simulink model "satelliteACModel"  (R2024a)
settings: Solver=ode45  StartTime=0.0  StopTime=800  MaxStep=1  RelTol=1e-8  AbsTol=1e-10
undefined symbols (not defined in the file or in its folder): Cw, Cwp, J, Kaw, Kd, Ki, Kp, r0, Td, Tmax, w0, x0, z0
settings Model: Creator=taole  LastModifiedBy=taole

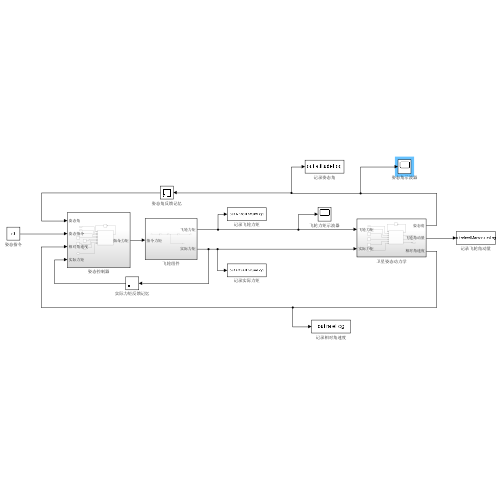
[thumbnail: Simulink's stored preview of the top-level diagram]
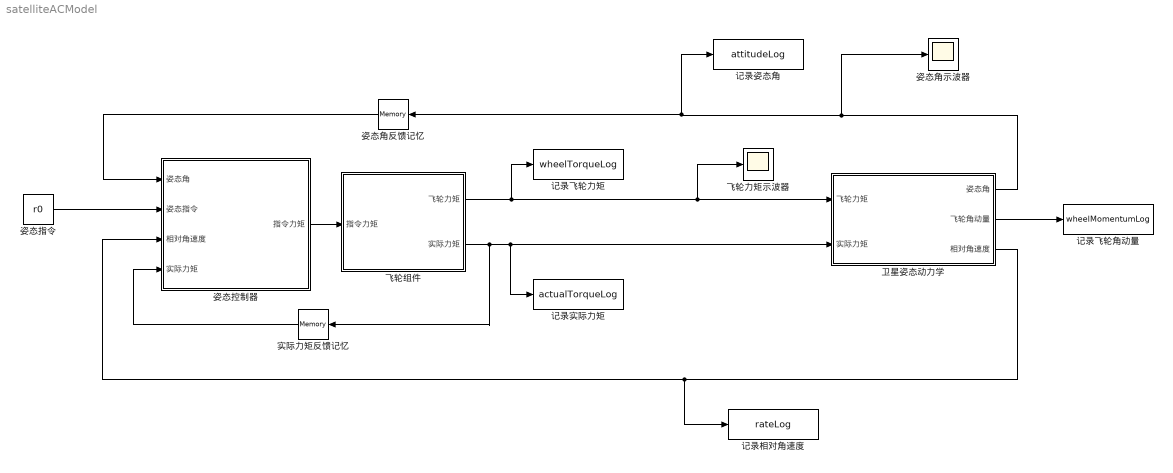
== system satelliteACModel ==
  卫星姿态动力学 : Subsystem
  姿态指令 : Constant  Value=r0
  姿态控制器 : Subsystem
  姿态角反馈记忆 : Memory  InitialCondition=[0;0;0]
  姿态角示波器 : Scope
  实际力矩反馈记忆 : Memory  InitialCondition=[0;0;0]
  记录姿态角 : ToWorkspace  VariableName=attitudeLog  SaveFormat=Structure With Time  SampleTime=-1
  记录实际力矩 : ToWorkspace  VariableName=actualTorqueLog  SaveFormat=Structure With Time  SampleTime=-1
  记录相对角速度 : ToWorkspace  VariableName=rateLog  SaveFormat=Structure With Time  SampleTime=-1
  记录飞轮力矩 : ToWorkspace  VariableName=wheelTorqueLog  SaveFormat=Structure With Time  SampleTime=-1
  记录飞轮角动量 : ToWorkspace  VariableName=wheelMomentumLog  SaveFormat=Structure With Time  SampleTime=-1
  飞轮力矩示波器 : Scope
  飞轮组件 : Subsystem
  wires:
  姿态控制器/1(指令力矩) -> 飞轮组件/1(指令力矩)
  飞轮组件/1(飞轮力矩) -> 记录飞轮力矩/1, 飞轮力矩示波器/1, 卫星姿态动力学/1(飞轮力矩)
  飞轮组件/2(实际力矩) -> 实际力矩反馈记忆/1, 记录实际力矩/1, 卫星姿态动力学/2(实际力矩)
  卫星姿态动力学/1(姿态角) -> 姿态角示波器/1, 记录姿态角/1, 姿态角反馈记忆/1
  卫星姿态动力学/3(相对角速度) -> 记录相对角速度/1, 姿态控制器/3(相对角速度)
  姿态指令/1 -> 姿态控制器/2(姿态指令)
  卫星姿态动力学/2(飞轮角动量) -> 记录飞轮角动量/1
  姿态角反馈记忆/1 -> 姿态控制器/1(姿态角)
  实际力矩反馈记忆/1 -> 姿态控制器/4(实际力矩)

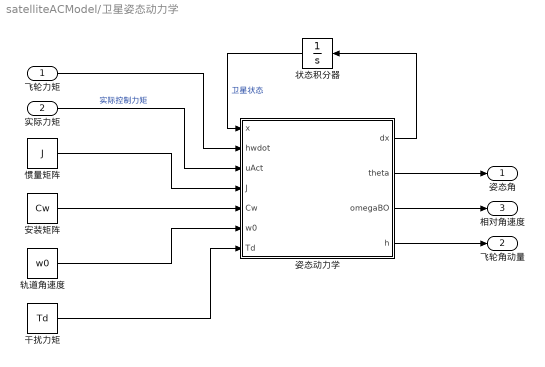
== system satelliteACModel/卫星姿态动力学 ==
  飞轮力矩 : Inport
  实际力矩 : Inport  Port=2
  姿态动力学 : MATLAB Function  TreatAsAtomicUnit=on
  安装矩阵 : Constant  Value=Cw
  干扰力矩 : Constant  Value=Td
  惯量矩阵 : Constant  Value=J
  状态积分器 : Integrator  InitialCondition=x0
  轨道角速度 : Constant  Value=w0
  姿态角 : Outport
  飞轮角动量 : Outport  Port=2
  相对角速度 : Outport  Port=3
  wires:
  姿态动力学/1(dx) -> 状态积分器/1
  状态积分器/1 -> 姿态动力学/1(x)  "卫星状态"
  飞轮力矩/1 -> 姿态动力学/2(hwdot)
  实际力矩/1 -> 姿态动力学/3(uAct)  "实际控制力矩"
  惯量矩阵/1 -> 姿态动力学/4(J)
  安装矩阵/1 -> 姿态动力学/5(Cw)
  轨道角速度/1 -> 姿态动力学/6(w0)
  干扰力矩/1 -> 姿态动力学/7(Td)
  姿态动力学/2(theta) -> 姿态角/1
  姿态动力学/3(omegaBO) -> 相对角速度/1
  姿态动力学/4(h) -> 飞轮角动量/1

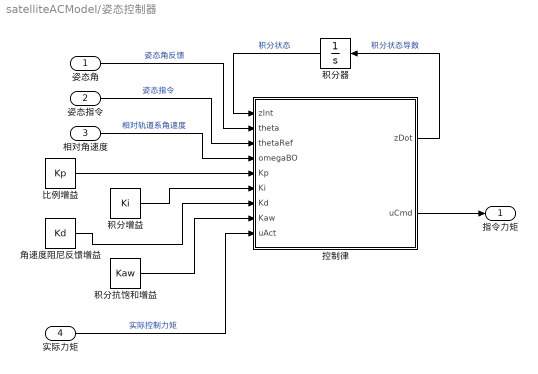
== system satelliteACModel/姿态控制器 ==
  姿态角 : Inport
  姿态指令 : Inport  Port=2
  相对角速度 : Inport  Port=3
  实际力矩 : Inport  Port=4
  控制律 : MATLAB Function  TreatAsAtomicUnit=on
  比例增益 : Constant  Value=Kp
  积分器 : Integrator  InitialCondition=z0
  积分增益 : Constant  Value=Ki
  积分抗饱和增益 : Constant  Value=Kaw
  角速度阻尼反馈增益 : Constant  Value=Kd
  指令力矩 : Outport
  wires:
  姿态指令/1 -> 控制律/3(thetaRef)  "姿态指令"
  姿态角/1 -> 控制律/2(theta)  "姿态角反馈"
  相对角速度/1 -> 控制律/4(omegaBO)  "相对轨道系角速度"
  比例增益/1 -> 控制律/5(Kp)
  积分增益/1 -> 控制律/6(Ki)
  角速度阻尼反馈增益/1 -> 控制律/7(Kd)
  积分抗饱和增益/1 -> 控制律/8(Kaw)
  控制律/1(zDot) -> 积分器/1  "积分状态导数"
  积分器/1 -> 控制律/1(zInt)  "积分状态"
  实际力矩/1 -> 控制律/9(uAct)  "实际控制力矩"
  控制律/2(uCmd) -> 指令力矩/1

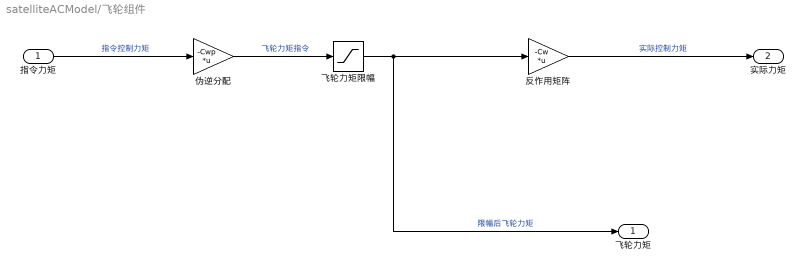
== system satelliteACModel/飞轮组件 ==
  指令力矩 : Inport
  伪逆分配 : Gain  Gain=-Cwp  Multiplication=Matrix(K*u)
  反作用矩阵 : Gain  Gain=-Cw  Multiplication=Matrix(K*u)
  飞轮力矩限幅 : Saturate  UpperLimit=Tmax*ones(4,1)  LowerLimit=-Tmax*ones(4,1)
  飞轮力矩 : Outport
  实际力矩 : Outport  Port=2
  wires:
  指令力矩/1 -> 伪逆分配/1  "指令控制力矩"
  伪逆分配/1 -> 飞轮力矩限幅/1  "飞轮力矩指令"
  飞轮力矩限幅/1 -> 反作用矩阵/1, 飞轮力矩/1  "限幅后飞轮力矩"
  反作用矩阵/1 -> 实际力矩/1  "实际控制力矩"

== matlab function satelliteACModel/卫星姿态动力学/姿态动力学 ==
  data: x input; dx output; hwdot input; uAct input; J input; Cw input; w0 input; Td input; theta output; omegaBO output; h output
function [dx, theta, omegaBO, h] = fcn(x, hwdot, uAct, J, Cw, w0, Td)
%#codegen

phi = x(1);
pitch = x(2);
psi = x(3);

omega = x(4:6);
hw = x(7:10);

cphi = cos(phi);
sphi = sin(phi);
cth = cos(pitch);
sth = sin(pitch);
cps = cos(psi);
sps = sin(psi);

Rx = [1 0 0;
      0 cphi sphi;
      0 -sphi cphi];

Ry = [cth 0 -sth;
      0 1 0;
      sth 0 cth];

Rz = [cps sps 0;
      -sps cps 0;
      0 0 1];

Cbo = Ry*Rx*Rz;

omegaOrbitBody = Cbo*[0; -w0; 0];

omegaBO = omega - omegaOrbitBody;

B = [-cphi*sth, cth, 0;
      sphi, 0, 1;
      cphi*cth, sth, 0];

rate = B\omegaBO;

h = Cw*hw;

omegaDot = J\(uAct + Td - cross(omega, J*omega + h));

dx = [rate(2);
      rate(3);
      rate(1);
      omegaDot;
      hwdot];

theta = [phi; pitch; psi];

end

== matlab function satelliteACModel/姿态控制器/控制律 ==
  data: zInt input; theta input; thetaRef input; zDot output; omegaBO input; Kp input; Ki input; Kd input; Kaw input; uAct input; uCmd output
function [zDot, uCmd] = fcn( zInt,  theta,thetaRef, omegaBO, Kp, Ki, Kd, Kaw, uAct)
%#codegen
% 姿态控制律：三轴 PID + back-calculation 抗积分饱和
%
% 输入变量说明：
% thetaRef : 姿态角指令，3×1，期望滚动角、俯仰角、偏航角
% theta    : 当前姿态角，3×1，当前滚动角、俯仰角、偏航角
% omegaBO  : 相对轨道系角速度，3×1，用作阻尼反馈
% zInt     : 积分状态，3×1，对姿态角误差积分
% uAct     : 实际控制力矩，3×1，飞轮限幅后反馈回来的体轴力矩
% Kp       : 比例增益，3×1
% Ki       : 积分增益，3×1
% Kd       : 阻尼增益，3×1
% Kaw      : 抗积分饱和增益，3×1
%
% 输出变量说明：
% zDot     : 积分状态导数，3×1
% uCmd     : 指令控制力矩，3×1，送入飞轮分配模块

% 姿态角误差
attitudeError = thetaRef - theta;

% PID 控制力矩
% 比例项：Kp * 姿态误差
% 积分项：Ki * 积分状态
% 阻尼项：-Kd * 相对角速度
uCmd = Kp(:).*attitudeError ...
     + Ki(:).*zInt ...
     - Kd(:).*omegaBO;

% 积分状态更新
% 第一项 attitudeError 是正常积分项
% 第二项 Kaw*(uAct-uCmd) 是抗积分饱和修正项
zDot = attitudeError ...
     + Kaw(:).*(uAct - uCmd);

end
